simulink model "smith_predictor_process"  (Simulink 3.00)
libraries: mathlib x2, modellib x1

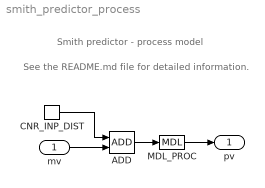
== system smith_predictor_process ==
  note: See the README.md file for detailed information.
  note: Smith predictor - process model
  mv : Inport  Port=1
  ADD : mathlib/ADD
  CNR_INP_DIST : mathlib/CNR  ycn=0
  MDL_PROC : modellib/MDL  k0=2  del=5  tau1=3  tau2=5  nmax=100
  pv : Outport  Port=1  nmax=100
  wires:
  ADD/1 -> MDL_PROC/1
  CNR_INP_DIST/1 -> ADD/1
  MDL_PROC/1 -> pv/1
  mv/1 -> ADD/2
